simulink library "elvio"  (R2017a)
settings: Solver=VariableStepAuto  StartTime=0.0  StopTime=10.0  RelTol=1e-3
values from neighbouring files (symbols this model uses):
  Ts = 1    [dynorun.m]
  v = squeeze(v)'    [elvio_plot_scatter.m]
undefined symbols (not defined in the file or in its folder): dm, energy, F, Fmax, Fmin, Freq, m, magnitude, vcur, vref
undefined symbols (not defined in the file): containers
libraries: elvio x38, simulink x6
settings Model: Creator=elts2  LastModifiedBy=thomas

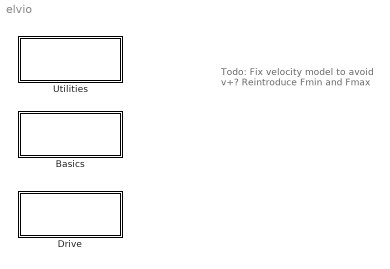
== system elvio ==
  note: Todo:
      | Fix velocity model to avoid v+?
      | Reintroduce Fmin and Fmax
  Basics : Subsystem
  Drive : Subsystem
  Utilities : Subsystem

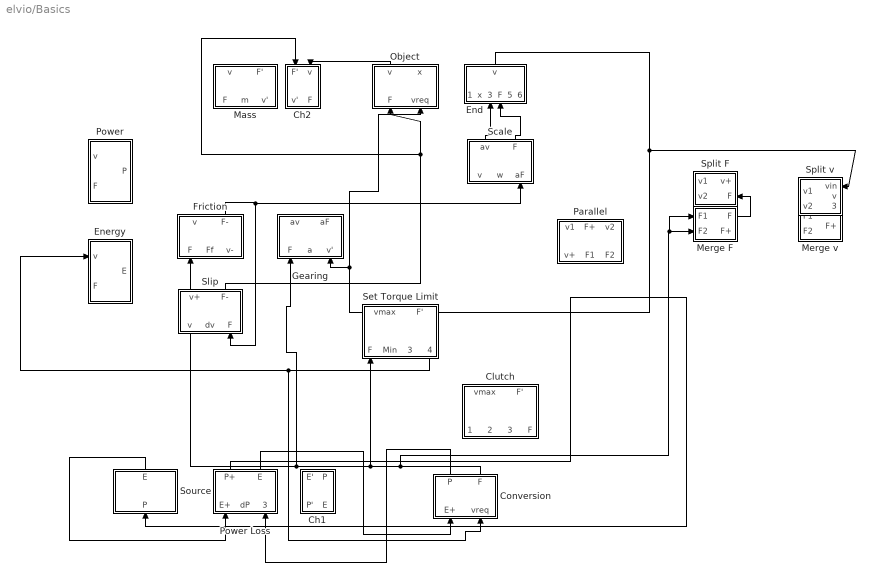
== system elvio/Basics ==
  Ch1 : Subsystem
  Ch2 : Subsystem
  Clutch : Subsystem
  Conversion : Subsystem
  End : Subsystem
  Energy : Subsystem
  Friction : Subsystem
  Gearing : Subsystem
  Mass : Subsystem
  Merge F : Subsystem
  Merge v : Subsystem
  Object : Subsystem
  Parallel : Subsystem
  Power : Subsystem
  Power Loss : Subsystem
  Scale : Subsystem
  Set Torque Limit : Subsystem
  Slip : Subsystem
  Source : Subsystem
  Split F : Subsystem
  Split v : Subsystem
  wires:
  Conversion/1(P) -> Power Loss/3(Preq)
  End/1(v) -> Split v/1(vin), Conversion/2(vreq), Energy/1(v), Object/2(vreq), Gearing/3(v')
  Power Loss/1(P+) -> Source/1(P)
  Source/1(E) -> Power Loss/1(E+)
  Conversion/2(F) -> Merge F/1(F1), Merge F/2(F2), Set Torque Limit/1(F), Gearing/1(F), Friction/1(F)
  Friction/2(F-) -> Scale/3(aF), Slip/3(F)
  Scale/1(av) -> End/3(vcur)
  Scale/2(F) -> End/4(F)
  Slip/2(F-) -> Ch2/1(F'), Object/1(F)
  Merge F/1(F) -> Split F/2(F)
  Power Loss/2(E) -> Conversion/1(E+)
  Object/1(v) -> Ch2/2(v)

== system elvio/Drive ==
  Engine : Subsystem  mask{Tmax=[40 50 60 80 100 120 150 200 300 500], Tmin=0, Tfrict=10, Ploss=1000, eff=0}
      mask prompts: Tmax "Max Torque:"; Tmin "Min Torque:"; Tfrict "Friction Torque:"; Ploss "Power Loss:"; eff "Efficiency:"
  Vehicle : Subsystem  mask{m=1200, Froll=15, Aeff=0.4, Tbrake=5000, n=[10 1]}
      mask prompts: m "Vehicle Mass:"; Froll "Tyre Friction:"; Aeff "Aero Drag:"; Tbrake "Braking Torque:"; n "Number of Simulation:"

== system elvio/Utilities ==
  Datafunction : Subsystem  mask{Cycle=NEDC, Data=[0 0 10 10 0 0]}
      mask prompts: Cycle "Driving Cycle:"; Data "Time Data:"
      mask init:
      | c=get_param(gcbh,'Cycle');
      | if c == "NEDC"
      |     set_param(gcbh,'Data','[0 0 10 10 0 0]');
      | end
      mask TypeOptions Cycle: NEDC | Artemis | FTP-75
  Display : Subsystem  StartFcn=h=add_exec_event_listener([gcb '/Display'], 'PostOutputs', @(blk,ev)set_param(gcbh,'MaskDisplay',['disp(''' num2str(blk.InputPort(1).Data) ''')']));  mask(Display the Input Value){}
      mask help: Todo: may display in the wrong blob? BUG
  Integrator : Subsystem  mask{Ts=Ts}
      mask prompts: Ts "Time Step:"
  Range : Subsystem
  Unit : Subsystem  mask(Constant value with units){Value=10, unitstr=rpm, unitmap=containers.Map({'rad/s','Hz','rpm','hrpm','krpm'},[1 2*pi 2*pi/60 2*pi/60*100 2*pi/60*1000])}
      mask prompts: Value "Simulink:blkprm_prompts:ConstConstValue"; unitmap "Unit map:"
      mask help:
      | This is a generic block for a value with units.
      |
      | The units can be configured with the field unitmap.
      mask TypeOptions Value: Constant/Value
      mask Display: disp('Value')
  Variants : Subsystem  Variant=on  VariantControl=Variant1  OverrideUsingVariant=Variant1

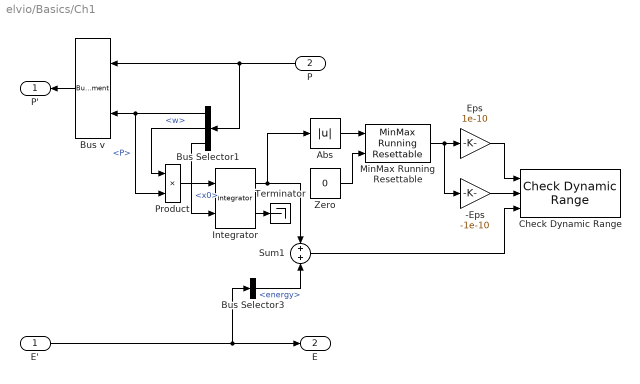
== system elvio/Basics/Ch1 ==
  E' : Inport
  P : Inport  Port=2
  -Eps : Gain  Gain=-1e-10
  Abs : Abs  ZeroCross=off
  Bus Selector1 : BusSelector  OutputSignals=P,info.w,info.x0
  Bus Selector3 : BusSelector  OutputSignals=energy
  Bus v : BusAssignment  AssignedSignals=P
  Check Dynamic Range : simulink/Model Verification/Check  Dynamic Range  Description=min < u < max  enabled=on  stopWhenAssertionFail=on  export=off  icon=graphic
      settings: SourceProductName=Simulink  SourceProductBaseCode=SL
  Eps : Gain  Gain=1e-10
  Integrator : elvio/Utilities/Integrator  Ts=Ts
  MinMax Running Resettable : simulink/Math Operations/MinMax Running Resettable  Function=max  vinit=1e-6
  Product : Product
  Sum1 : Sum
  Terminator : Terminator
  Zero : Constant  Value=0
  P' : Outport
  E : Outport  Port=2
  wires:
  Product/1 -> Integrator/1
  Bus Selector3/1 -> Sum1/2  "<energy>"
  E'/1 -> E/1, Bus Selector3/1
  Bus Selector1/3 -> Integrator/2  "<x0>"
  P/1 -> Bus Selector1/1, Bus v/1
  Bus Selector1/1 -> Bus v/2, Product/2  "<P>"
  Bus v/1 -> P'/1
  Bus Selector1/2 -> Product/1  "<w>"
  Integrator/2 -> Terminator/1
  Integrator/1 -> Abs/1, Sum1/1
  Sum1/1 -> Check Dynamic Range/3
  -Eps/1 -> Check Dynamic Range/2
  MinMax Running Resettable/1 -> -Eps/1, Eps/1
  Eps/1 -> Check Dynamic Range/1
  Zero/1 -> MinMax Running Resettable/2
  Abs/1 -> MinMax Running Resettable/1

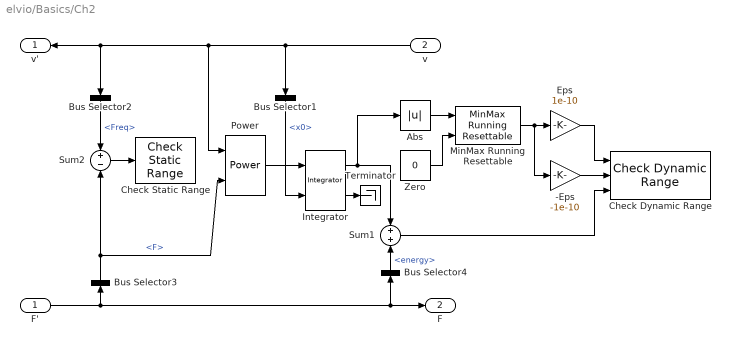
== system elvio/Basics/Ch2 ==
  F' : Inport
  v : Inport  Port=2
  -Eps : Gain  Gain=-1e-10
  Abs : Abs  ZeroCross=off
  Bus Selector1 : BusSelector  OutputSignals=info.x0
  Bus Selector2 : BusSelector  OutputSignals=Freq
  Bus Selector3 : BusSelector  OutputSignals=F
  Bus Selector4 : BusSelector  OutputSignals=energy
  Check Dynamic Range : simulink/Model Verification/Check  Dynamic Range  Description=min < u < max  enabled=on  stopWhenAssertionFail=on  export=off  icon=graphic
      settings: SourceProductName=Simulink  SourceProductBaseCode=SL
  Check Static Range : simulink/Model Verification/Check  Static Range  Description=-1e-10 <= u <= 1e-10  max=1e-10  max_included=on  min=-1e-10  min_included=on  enabled=on  stopWhenAssertionFail=on  export=off  icon=graphic
      settings: SourceProductName=Simulink  SourceProductBaseCode=SL
  Eps : Gain  Gain=1e-10
  Integrator : elvio/Utilities/Integrator  Ts=Ts
  MinMax Running Resettable : simulink/Math Operations/MinMax Running Resettable  Function=max  vinit=1e-6
  Power : elvio/Basics/Power
  Sum1 : Sum
  Sum2 : Sum  Inputs=+-
  Terminator : Terminator
  Zero : Constant  Value=0
  v' : Outport
  F : Outport  Port=2
  wires:
  Bus Selector3/1 -> Power/2, Sum2/2  "<F>"
  -Eps/1 -> Check Dynamic Range/2
  MinMax Running Resettable/1 -> -Eps/1, Eps/1
  Eps/1 -> Check Dynamic Range/1
  Abs/1 -> MinMax Running Resettable/1
  Power/1 -> Integrator/1
  Sum1/1 -> Check Dynamic Range/3
  Bus Selector4/1 -> Sum1/2  "<energy>"
  F'/1 -> F/1, Bus Selector4/1, Bus Selector3/1
  Bus Selector1/1 -> Integrator/2  "<x0>"
  v/1 -> Bus Selector1/1, Power/1, Bus Selector2/1, v'/1
  Integrator/2 -> Terminator/1
  Integrator/1 -> Sum1/1, Abs/1
  Zero/1 -> MinMax Running Resettable/2
  Bus Selector2/1 -> Sum2/1  "<Freq>"
  Sum2/1 -> Check Static Range/1

== system elvio/Basics/Clutch ==
  note: Todo
  vreq : Inport
  Fmax : Inport  Port=2
  Fmin : Inport  Port=3
  F : Inport  Port=4
  Bus Selector1 : BusSelector  OutputSignals=Freq
  Bus F : BusAssignment  AssignedSignals=Fmax,Fmin,F
  Bus v : BusAssignment  AssignedSignals=Freq
  Range : Subsystem
  vmax : Outport
  F' : Outport  Port=2
  wires:
  F/1 -> Bus F/1
  Range/1(Out) -> Bus F/4, Bus v/2  "F"
  Bus Selector1/1 -> Range/2(In)  "<Freq>"
  vreq/1 -> Bus v/1, Bus Selector1/1
  Bus v/1 -> vmax/1
  Fmin/1 -> Range/3(Min), Bus F/3  "Fmin"
  Fmax/1 -> Range/1(Max), Bus F/2
  Bus F/1 -> F'/1

== system elvio/Basics/Conversion ==
  E+ : Inport
  vreq : Inport  Port=2
  Bias1 : Bias  Bias=1e10
  Bias2 : Bias  Bias=-1e10
  Bus Creator1 : BusCreator  Inputs=8
  Bus Selector : BusSelector  OutputSignals=info.x0,Freq
  Bus Selector3 : BusSelector  OutputSignals=energy
  Constant{4..7} (4 alike) : Constant  Value=0
  Power : Subsystem
  unity : Gain
  zero : Gain  Gain=0
  P : Outport
  F : Outport  Port=2
  wires:
  Power/1(P) -> P/1
  Constant7/1 -> Bus Creator1/7  "power"
  Constant5/1 -> Bus Creator1/5  "dm"
  Bus Selector/2 -> unity/1, Power/2(F)  "<Freq>"
  Bus Creator1/1 -> F/1
  Constant6/1 -> Bus Creator1/6  "weight"
  Constant4/1 -> Bus Creator1/4  "m"
  vreq/1 -> Power/1(v), Bus Selector/1
  unity/1 -> Bus Creator1/1  "F"
  E+/1 -> Bus Selector3/1
  Bus Selector3/1 -> Bus Creator1/8  "<energy>"
  zero/1 -> Bias2/1, Bias1/1
  Bias2/1 -> Bus Creator1/3  "Fmin"
  Bus Selector/1 -> zero/1  "<x0>"
  Bias1/1 -> Bus Creator1/2  "Fmax"

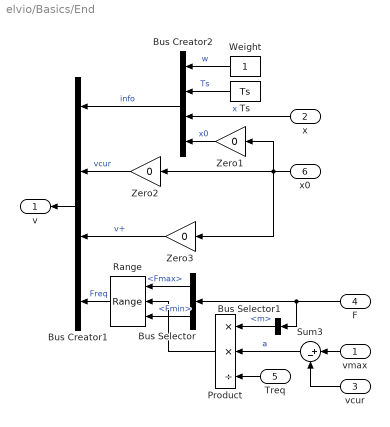
== system elvio/Basics/End ==
  vmax : Inport  Unit=m/s
  x : Inport  Port=2  Unit=m/s
  vcur : Inport  Port=3  Unit=m/s
  F : Inport  Port=4  Unit=m/s
  Treq : Inport  Port=5  Unit=m/s
  x0 : Inport  Port=6  Unit=m/s
  Bus Creator1 : BusCreator  Inputs=4
  Bus Creator2 : BusCreator  Inputs=4
  Bus Selector : BusSelector  OutputSignals=Fmax,Fmin
  Bus Selector1 : BusSelector  OutputSignals=m
  Product : Product  Inputs=**/
  Range : elvio/Utilities/Range
  Sum3 : Sum  Inputs=|+-
  Ts : Constant  Value=Ts
  Weight : Constant
  Zero1 : Gain  Gain=0
  Zero2 : Gain  Gain=0
  Zero3 : Gain  Gain=0
  v : Outport
  wires:
  x/1 -> Bus Creator2/3  "x"
  Weight/1 -> Bus Creator2/1  "w"
  Bus Creator1/1 -> v/1
  vmax/1 -> Sum3/1
  F/1 -> Bus Selector/1, Bus Selector1/1
  Bus Creator2/1 -> Bus Creator1/1  "info"
  Range/1 -> Bus Creator1/4  "Freq"
  Sum3/1 -> Product/2  "a"
  Zero2/1 -> Bus Creator1/2  "vcur"
  Zero3/1 -> Bus Creator1/3  "v+"
  vcur/1 -> Sum3/2
  Treq/1 -> Product/3
  x0/1 -> Zero2/1, Zero3/1, Zero1/1
  Zero1/1 -> Bus Creator2/4  "x0"
  Ts/1 -> Bus Creator2/2  "Ts"
  Bus Selector1/1 -> Product/1  "<m>"
  Bus Selector/1 -> Range/1  "<Fmax>"
  Bus Selector/2 -> Range/3  "<Fmin>"
  Product/1 -> Range/2

== system elvio/Basics/Energy ==
  v : Inport
  F : Inport  Port=2
  Bus Selector : BusSelector  OutputSignals=info.x0
  Integrator : elvio/Utilities/Integrator
  Power : elvio/Basics/Power
  Terminator : Terminator
  E : Outport
  wires:
  v/1 -> Bus Selector/1, Power/1
  Power/1 -> Integrator/1
  F/1 -> Power/2
  Bus Selector/1 -> Integrator/2  "<x0>"
  Integrator/2 -> Terminator/1
  Integrator/1 -> E/1

== system elvio/Basics/Friction ==
  F : Inport
  Ff : Inport  Port=2
  v- : Inport  Port=3
  Bus Selector : BusSelector  OutputSignals=F,Fmax,Fmin,energy
  Bus Selector1 : BusSelector  OutputSignals=Freq
  Bus F : BusAssignment  AssignedSignals=F,Fmax,Fmin,energy
  Bus v : BusAssignment  AssignedSignals=Freq
  Display : Display
  Energy : elvio/Basics/Energy
  Sum1 : Sum  Inputs=++|
  Sum2 : Sum  Inputs=-+|
  Sum3 : Sum  Inputs=|++
  Sum4 : Sum  Inputs=-+|
  Sum5 : Sum  Inputs=-+|
  v : Outport
  F- : Outport  Port=2
  wires:
  Energy/1 -> Display/1, Sum1/1  "E_loss_fric"
  v-/1 -> Energy/1, Bus Selector1/1, Bus v/1
  Sum3/1 -> Bus v/2  "Freq"
  Bus Selector1/1 -> Sum3/1  "<Freq>"
  Sum2/1 -> Bus F/2  "F"
  Bus F/1 -> F-/1
  Ff/1 -> Sum4/1, Sum5/1, Energy/2, Sum2/1, Sum3/2
  Bus v/1 -> v/1
  F/1 -> Bus Selector/1, Bus F/1
  Bus Selector/1 -> Sum2/2  "<F>"
  Sum1/1 -> Bus F/5
  Bus Selector/4 -> Sum1/2  "<energy>"
  Bus Selector/2 -> Sum4/2  "<Fmax>"
  Bus Selector/3 -> Sum5/2  "<Fmin>"
  Sum5/1 -> Bus F/4  "Fmin"
  Sum4/1 -> Bus F/3  "Fmax"

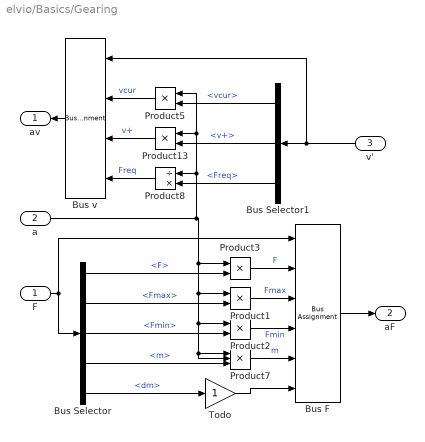
== system elvio/Basics/Gearing ==
  F : Inport
  a : Inport  Port=2
  v' : Inport  Port=3
  Bus Selector : BusSelector  OutputSignals=F,Fmax,Fmin,m,dm
  Bus Selector1 : BusSelector  OutputSignals=vcur,v+,Freq
  Bus F : BusAssignment  AssignedSignals=F,Fmax,Fmin,m,dm
  Bus v : BusAssignment  AssignedSignals=vcur,v+,Freq
  Product{1..3,5,13} (5 alike) : Product
  Product7 : Product  Inputs=***
  Product8 : Product  Inputs=/*
  Todo : Gain
  av : Outport
  aF : Outport  Port=2
  wires:
  Bus F/1 -> aF/1
  Todo/1 -> Bus F/6
  v'/1 -> Bus Selector1/1, Bus v/1
  Bus Selector1/2 -> Product13/2  "<v+>"
  Product13/1 -> Bus v/3  "v+"
  Bus Selector1/1 -> Product5/2  "<vcur>"
  F/1 -> Bus Selector/1, Bus F/1
  Product8/1 -> Bus v/4  "Freq"
  Bus v/1 -> av/1
  Bus Selector/5 -> Todo/1  "<dm>"
  Bus Selector/1 -> Product3/2  "<F>"
  Bus Selector/4 -> Product7/3  "<m>"
  a/1 -> Product8/1, Product5/1, Product13/1, Product1/1, Product2/1, Product7/2, Product7/1, Product3/1
  Product7/1 -> Bus F/5  "m"
  Product3/1 -> Bus F/2  "F"
  Bus Selector1/3 -> Product8/2  "<Freq>"
  Product5/1 -> Bus v/2  "vcur"
  Product1/1 -> Bus F/3  "Fmax"
  Bus Selector/2 -> Product1/2  "<Fmax>"
  Product2/1 -> Bus F/4  "Fmin"
  Bus Selector/3 -> Product2/2  "<Fmin>"

== system elvio/Basics/Mass ==
  F : Inport
  m : Inport  Port=2
  v' : Inport  Port=3
  Bus Assignment : BusAssignment  AssignedSignals=m
  Bus Selector : BusSelector  OutputSignals=m
  Sum : Sum  Inputs=|++
  v : Outport
  F' : Outport  Port=2
  wires:
  m/1 -> Sum/2
  Sum/1 -> Bus Assignment/2  "m"
  Bus Selector/1 -> Sum/1  "<m>"
  v'/1 -> v/1
  F/1 -> Bus Assignment/1, Bus Selector/1
  Bus Assignment/1 -> F'/1

== system elvio/Basics/Merge F ==
  F1 : Inport
  F2 : Inport  Port=2
  Bus Creator : BusCreator  Inputs=8
  Bus Selector : BusSelector  OutputSignals=F,Fmax,Fmin,m,dm,weight,power,energy
  Bus Selector2 : BusSelector  OutputSignals=F,Fmax,Fmin,m,dm,weight,power,energy
  Sum{,1..7} (8 alike) : Sum  Inputs=|++
  F : Outport
  F+ : Outport  Port=2
  wires:
  Bus Selector/6 -> Sum3/1  "<weight>"
  Bus Selector/4 -> Sum1/1  "<m>"
  Bus Selector/5 -> Sum2/1  "<dm>"
  Bus Selector/7 -> Sum4/1  "<power>"
  F1/1 -> Bus Selector/1, F/1
  Bus Selector/1 -> Sum/1  "<F>"
  F2/1 -> Bus Selector2/1
  Bus Creator/1 -> F+/1
  Sum/1 -> Bus Creator/1  "F"
  Sum2/1 -> Bus Creator/5  "dm"
  Bus Selector2/5 -> Sum2/2  "<dm>"
  Bus Selector2/1 -> Sum/2  "<F>"
  Bus Selector2/7 -> Sum4/2  "<power>"
  Sum4/1 -> Bus Creator/7  "power"
  Sum6/1 -> Bus Creator/8  "energy"
  Sum1/1 -> Bus Creator/4  "m"
  Sum3/1 -> Bus Creator/6  "weight"
  Bus Selector/8 -> Sum6/1  "<energy>"
  Bus Selector2/6 -> Sum3/2  "<weight>"
  Bus Selector2/8 -> Sum6/2  "<energy>"
  Bus Selector2/4 -> Sum1/2  "<m>"
  Bus Selector/3 -> Sum7/1  "<Fmin>"
  Sum7/1 -> Bus Creator/3  "Fmin"
  Bus Selector/2 -> Sum5/1  "<Fmax>"
  Sum5/1 -> Bus Creator/2  "Fmax"
  Bus Selector2/2 -> Sum5/2  "<Fmax>"
  Bus Selector2/3 -> Sum7/2  "<Fmin>"

== system elvio/Basics/Merge v ==
  note: Todo
  F1 : Inport
  F2 : Inport  Port=2
  Bus Creator : BusCreator  Inputs=8
  Bus Selector : BusSelector  OutputSignals=F,Fmax,Fmin,m,dm,weight,power,energy
  Bus Selector2 : BusSelector  OutputSignals=F,Fmax,Fmin,m,dm,weight,power,energy
  Highest Min : MinMax  Function=max  Inputs=2
  Lowest Max : MinMax  Inputs=2
  Sum{1..4,6} (5 alike) : Sum  Inputs=|++
  F+ : Outport
  wires:
  Bus Selector2/3 -> Highest Min/2  "<Fmin>"
  Bus Selector2/2 -> Lowest Max/2  "<Fmax>"
  Lowest Max/1 -> Bus Creator/2  "Fmax"
  Bus Selector/2 -> Lowest Max/1  "<Fmax>"
  Highest Min/1 -> Bus Creator/3  "Fmin"
  Bus Selector/3 -> Highest Min/1  "<Fmin>"
  Bus Selector2/4 -> Sum1/2  "<m>"
  Bus Selector2/8 -> Sum6/2  "<energy>"
  Bus Selector2/6 -> Sum3/2  "<weight>"
  Bus Selector/8 -> Sum6/1  "<energy>"
  Sum3/1 -> Bus Creator/6  "weight"
  Sum1/1 -> Bus Creator/4  "m"
  Sum6/1 -> Bus Creator/8  "energy"
  Sum4/1 -> Bus Creator/7  "power"
  Bus Selector2/7 -> Sum4/2  "<power>"
  Bus Selector2/5 -> Sum2/2  "<dm>"
  Sum2/1 -> Bus Creator/5  "dm"
  Bus Creator/1 -> F+/1
  F2/1 -> Bus Selector2/1
  Bus Selector/1 -> Bus Creator/1  "<F>"
  F1/1 -> Bus Selector/1
  Bus Selector/7 -> Sum4/1  "<power>"
  Bus Selector/5 -> Sum2/1  "<dm>"
  Bus Selector/4 -> Sum1/1  "<m>"
  Bus Selector/6 -> Sum3/1  "<weight>"

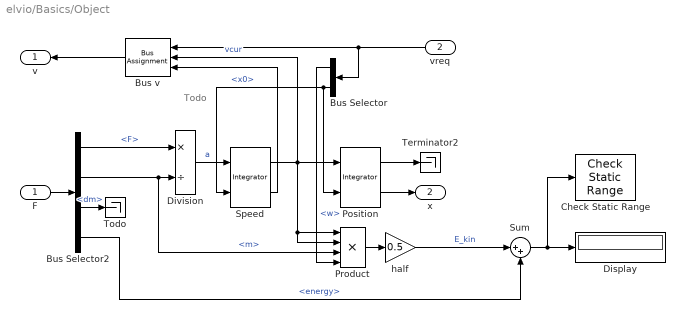
== system elvio/Basics/Object ==
  note: Todo
  F : Inport
  vreq : Inport  Port=2
  Bus Selector : BusSelector  OutputSignals=info.w,info.x0
  Bus Selector2 : BusSelector  OutputSignals=F,m,dm,energy
  Bus v : BusAssignment  AssignedSignals=vcur,v+
  Check Static Range : simulink/Model Verification/Check  Static Range  Description=-1e-3 <= u <= 1e-3  max=1e-3  max_included=on  min=-1e-3  min_included=on  enabled=on  stopWhenAssertionFail=on  export=off  icon=graphic
      settings: SourceProductName=Simulink  SourceProductBaseCode=SL
  Display : Display
  Division : Product  Inputs=*/
  Position : elvio/Utilities/Integrator  Ts=Ts
  Product : Product  Inputs=****
  Speed : elvio/Utilities/Integrator  Ts=Ts
  Sum : Sum  Inputs=|++
  Terminator2 : Terminator
  Todo : Terminator
  half : Gain  Gain=0.5
  v : Outport
  x : Outport  Port=2
  wires:
  vreq/1 -> Bus Selector/1, Bus v/1
  Bus Selector2/2 -> Product/3, Division/2  "<m>"
  Speed/1 -> Position/1, Bus v/2, Product/2, Product/1  "vcur"
  Division/1 -> Speed/1  "a"
  Product/1 -> half/1
  Bus Selector2/1 -> Division/1  "<F>"
  F/1 -> Bus Selector2/1
  half/1 -> Sum/1  "E_kin"
  Bus Selector2/3 -> Todo/1  "<dm>"
  Bus v/1 -> v/1
  Bus Selector/1 -> Product/4  "<w>"
  Position/2 -> x/1
  Position/1 -> Terminator2/1
  Speed/2 -> Bus v/3
  Bus Selector/2 -> Position/2, Speed/2  "<x0>"
  Bus Selector2/4 -> Sum/2  "<energy>"
  Sum/1 -> Check Static Range/1, Display/1

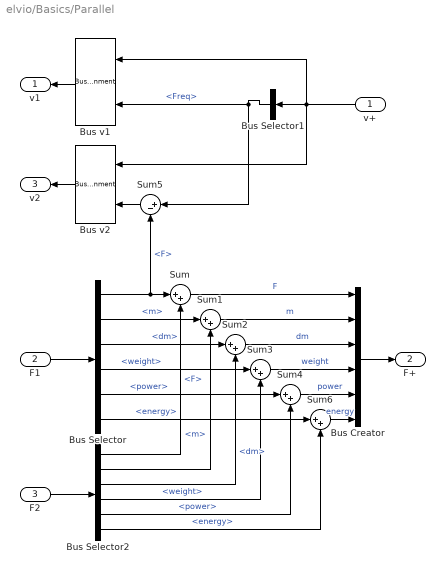
== system elvio/Basics/Parallel ==
  v+ : Inport
  F1 : Inport  Port=2
  F2 : Inport  Port=3
  Bus Creator : BusCreator  Inputs=6
  Bus Selector : BusSelector  OutputSignals=F,m,dm,weight,power,energy
  Bus Selector1 : BusSelector  OutputSignals=Freq
  Bus Selector2 : BusSelector  OutputSignals=F,m,dm,weight,power,energy
  Bus v1 : BusAssignment  AssignedSignals=Freq
  Bus v2 : BusAssignment  AssignedSignals=Freq
  Sum{,1..4,6} (6 alike) : Sum  Inputs=|++
  Sum5 : Sum  Inputs=|+-
  v1 : Outport
  F+ : Outport  Port=2
  v2 : Outport  Port=3
  wires:
  F1/1 -> Bus Selector/1
  Bus v1/1 -> v1/1
  Bus Selector1/1 -> Bus v1/2, Sum5/1  "<Freq>"
  Bus v2/1 -> v2/1
  v+/1 -> Bus v1/1, Bus v2/1, Bus Selector1/1
  Bus Selector/4 -> Sum3/1  "<weight>"
  Bus Selector/3 -> Sum2/1  "<dm>"
  Bus Selector/5 -> Sum4/1  "<power>"
  Bus Selector/2 -> Sum1/1  "<m>"
  Bus Selector/1 -> Sum5/2, Sum/1  "<F>"
  F2/1 -> Bus Selector2/1
  Bus Selector2/1 -> Sum/2  "<F>"
  Bus Selector2/2 -> Sum1/2  "<m>"
  Bus Selector2/3 -> Sum2/2  "<dm>"
  Bus Selector2/4 -> Sum3/2  "<weight>"
  Bus Selector2/5 -> Sum4/2  "<power>"
  Sum/1 -> Bus Creator/1  "F"
  Sum1/1 -> Bus Creator/2  "m"
  Sum2/1 -> Bus Creator/3  "dm"
  Sum3/1 -> Bus Creator/4  "weight"
  Sum4/1 -> Bus Creator/5  "power"
  Bus Creator/1 -> F+/1
  Sum5/1 -> Bus v2/2
  Sum6/1 -> Bus Creator/6  "energy"
  Bus Selector2/6 -> Sum6/2  "<energy>"
  Bus Selector/6 -> Sum6/1  "<energy>"

== system elvio/Basics/Power ==
  v : Inport
  F : Inport  Port=2
  Bus Selector2 : BusSelector  OutputSignals=vcur,v+,info.w
  Product : Product  Inputs=***
  Sum4 : Sum  Inputs=++|
  half : Gain  Gain=0.5
  P : Outport
  wires:
  half/1 -> P/1
  Bus Selector2/3 -> Product/2  "<w>"
  Bus Selector2/2 -> Sum4/2  "<v+>"
  Bus Selector2/1 -> Sum4/1  "<vcur>"
  F/1 -> Product/3
  v/1 -> Bus Selector2/1
  Sum4/1 -> Product/1
  Product/1 -> half/1

== system elvio/Basics/Power Loss ==
  E+ : Inport
  dP : Inport  Port=2
  Preq : Inport  Port=3
  Bus Selector1 : BusSelector  OutputSignals=P,info.w,info.x0
  Bus Selector3 : BusSelector  OutputSignals=energy
  Bus E : BusAssignment  AssignedSignals=energy
  Bus v : BusAssignment  AssignedSignals=P
  Display : Display
  Integrator : elvio/Utilities/Integrator  Ts=Ts
  Product : Product
  Sum1 : Sum  Inputs=++|
  Sum3 : Sum  Inputs=|++
  Terminator : Terminator
  P+ : Outport
  E : Outport  Port=2
  wires:
  Integrator/1 -> Sum1/1, Display/1  "E_power_loss"
  Integrator/2 -> Terminator/1
  Product/1 -> Integrator/1
  Bus Selector1/2 -> Product/1  "<w>"
  Bus v/1 -> P+/1
  Bus Selector1/1 -> Sum3/1  "<P>"
  Sum3/1 -> Bus v/2  "Freq"
  dP/1 -> Sum3/2, Product/2
  Preq/1 -> Bus v/1, Bus Selector1/1
  Bus Selector1/3 -> Integrator/2  "<x0>"
  E+/1 -> Bus Selector3/1, Bus E/1
  Sum1/1 -> Bus E/2
  Bus E/1 -> E/1
  Bus Selector3/1 -> Sum1/2  "<energy>"

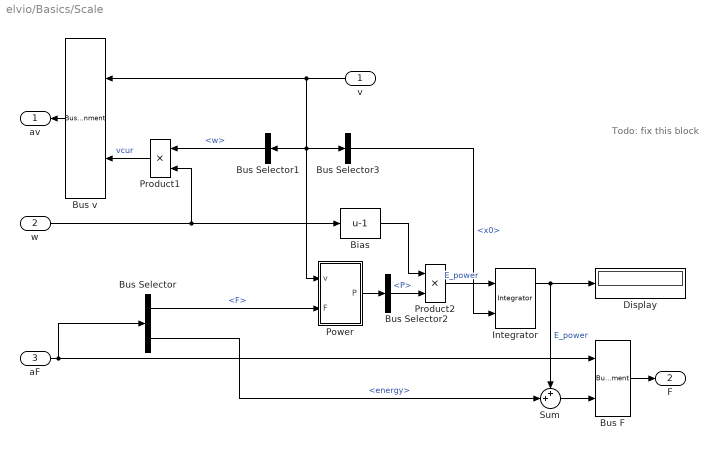
== system elvio/Basics/Scale ==
  note: Todo: fix this block
  v : Inport
  w : Inport  Port=2
  aF : Inport  Port=3
  Bias : Bias  Bias=-1
  Bus Selector : BusSelector  OutputSignals=F,energy
  Bus Selector1 : BusSelector  OutputSignals=info.w
  Bus Selector2 : BusSelector  OutputSignals=P
  Bus Selector3 : BusSelector  OutputSignals=info.x0
  Bus F : BusAssignment  AssignedSignals=energy
  Bus v : BusAssignment  AssignedSignals=info.w
  Display : Display
  Integrator : elvio/Utilities/Integrator  Ts=Ts
  Power : Subsystem
  Product1 : Product
  Product2 : Product
  Sum : Sum  Inputs=++|
  av : Outport
  F : Outport  Port=2
  wires:
  Integrator/1 -> Sum/1, Display/1  "E_power"
  Bus Selector3/1 -> Integrator/2  "<x0>"
  Product2/1 -> Integrator/1  "E_power"
  Bias/1 -> Product2/1
  w/1 -> Product1/2, Bias/1
  Bus Selector2/1 -> Product2/2  "<P>"
  Bus Selector/1 -> Power/2(F)  "<F>"
  v/1 -> Bus v/1, Bus Selector1/1, Power/1(v), Bus Selector3/1
  Power/1(P) -> Bus Selector2/1
  Product1/1 -> Bus v/2  "vcur"
  Bus v/1 -> av/1
  Bus Selector1/1 -> Product1/1  "<w>"
  aF/1 -> Bus Selector/1, Bus F/1
  Bus F/1 -> F/1
  Sum/1 -> Bus F/2
  Bus Selector/2 -> Sum/2  "<energy>"

== system elvio/Basics/Set Torque Limit ==
  F : Inport
  Min : Inport  Port=2
  Max : Inport  Port=3
  vreq : Inport  Port=4
  Bus Selector : BusSelector  OutputSignals=Freq
  Bus Selector1 : BusSelector  OutputSignals=Fmax,Fmin
  Bus F : BusAssignment  AssignedSignals=Fmax,Fmin
  Bus v : BusAssignment  AssignedSignals=Freq
  Highest Min : MinMax  Function=max  Inputs=2
  Lowest Max : MinMax  Inputs=2
  Range : elvio/Utilities/Range
  vmax : Outport
  F' : Outport  Port=2
  wires:
  F/1 -> Bus Selector1/1, Bus F/1
  Bus v/1 -> vmax/1
  vreq/1 -> Bus Selector/1, Bus v/1
  Range/1 -> Bus v/2
  Bus Selector/1 -> Range/2  "<Freq>"
  Bus F/1 -> F'/1
  Lowest Max/1 -> Range/1, Bus F/2
  Highest Min/1 -> Range/3, Bus F/3
  Bus Selector1/1 -> Lowest Max/2  "<Fmax>"
  Bus Selector1/2 -> Highest Min/2  "<Fmin>"
  Max/1 -> Lowest Max/1
  Min/1 -> Highest Min/1

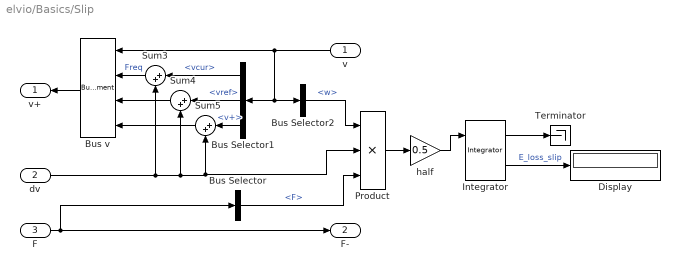
== system elvio/Basics/Slip ==
  v : Inport
  dv : Inport  Port=2
  F : Inport  Port=3
  Bus Selector : BusSelector  OutputSignals=F
  Bus Selector1 : BusSelector  OutputSignals=vcur,vref,v+
  Bus Selector2 : BusSelector  OutputSignals=info.w
  Bus v : BusAssignment  AssignedSignals=vcur,vref,v+
  Display : Display
  Integrator : elvio/Utilities/Integrator  Ts=Ts
  Product : Product  Inputs=***
  Sum3 : Sum  Inputs=|++
  Sum4 : Sum  Inputs=|++
  Sum5 : Sum  Inputs=|++
  Terminator : Terminator
  half : Gain  Gain=0.5
  v+ : Outport
  F- : Outport  Port=2
  wires:
  Bus Selector2/1 -> Product/1  "<w>"
  v/1 -> Bus v/1, Bus Selector1/1, Bus Selector2/1
  half/1 -> Integrator/1
  Bus Selector/1 -> Product/3  "<F>"
  Integrator/2 -> Display/1  "E_loss_slip"
  Product/1 -> half/1
  dv/1 -> Sum3/2, Sum5/2, Product/2, Sum4/2
  Integrator/1 -> Terminator/1
  Sum5/1 -> Bus v/4
  Bus Selector1/2 -> Sum4/1  "<vref>"
  Bus Selector1/3 -> Sum5/1  "<v+>"
  Sum4/1 -> Bus v/3
  Sum3/1 -> Bus v/2  "Freq"
  Bus Selector1/1 -> Sum3/1  "<vcur>"
  F/1 -> Bus Selector/1, F-/1
  Bus v/1 -> v+/1

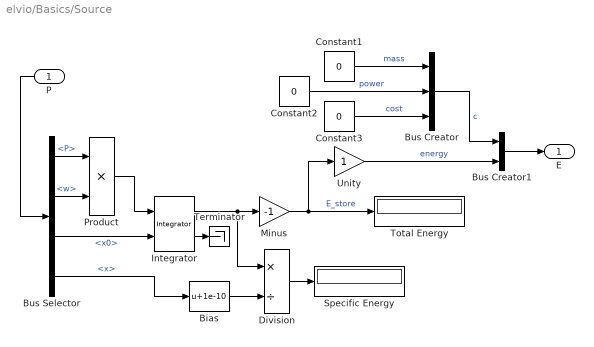
== system elvio/Basics/Source ==
  P : Inport
  Bias : Bias  Bias=1e-10
  Bus Creator : BusCreator  Inputs=3
  Bus Creator1 : BusCreator  Inputs=2
  Bus Selector : BusSelector  OutputSignals=P,info.w,info.x0,info.x
  Constant1 : Constant  Value=0
  Constant2 : Constant  Value=0
  Constant3 : Constant  Value=0
  Division : Product  Inputs=*/
  Integrator : elvio/Utilities/Integrator  Ts=Ts
  Minus : Gain  Gain=-1
  Product : Product  Inputs=**
  Specific Energy : Display
  Terminator : Terminator
  Total Energy : Display
  Unity : Gain
  E : Outport
  wires:
  Integrator/2 -> Terminator/1
  Minus/1 -> Unity/1, Total Energy/1  "E_store"
  Product/1 -> Integrator/1
  P/1 -> Bus Selector/1
  Bus Selector/1 -> Product/1  "<P>"
  Bus Selector/2 -> Product/2  "<w>"
  Bus Selector/4 -> Bias/1  "<x>"
  Division/1 -> Specific Energy/1
  Bus Selector/3 -> Integrator/2  "<x0>"
  Integrator/1 -> Minus/1, Division/1
  Unity/1 -> Bus Creator1/2  "energy"
  Bus Creator/1 -> Bus Creator1/1  "c"
  Bus Creator1/1 -> E/1
  Constant1/1 -> Bus Creator/1  "mass"
  Constant3/1 -> Bus Creator/3  "cost"
  Constant2/1 -> Bus Creator/2  "power"
  Bias/1 -> Division/2

== system elvio/Basics/Split F ==
  v+ : Inport
  F : Inport  Port=2
  Bus Selector : BusSelector  OutputSignals=F,Fmax,Fmin
  Bus Selector1 : BusSelector  OutputSignals=Freq
  Bus v1 : BusAssignment  AssignedSignals=Freq
  Bus v2 : BusAssignment  AssignedSignals=Freq
  Range : elvio/Utilities/Range
  Sum5 : Sum  Inputs=|+-
  v1 : Outport
  v2 : Outport  Port=2
  wires:
  Bus v2/1 -> v2/1
  Bus v1/1 -> v1/1
  Bus Selector1/1 -> Range/2, Sum5/1  "<Freq>"
  v+/1 -> Bus v2/1, Bus v1/1, Bus Selector1/1
  Sum5/1 -> Bus v2/2
  F/1 -> Bus Selector/1
  Bus Selector/1 -> Sum5/2  "<F>"
  Range/1 -> Bus v1/2
  Bus Selector/2 -> Range/1  "<Fmax>"
  Bus Selector/3 -> Range/3  "<Fmin>"

== system elvio/Basics/Split v ==
  vin : Inport
  v : Inport  Port=2
  v+1 : Inport  Port=3
  Bus Selector1 : BusSelector  OutputSignals=vcur,v+
  Bus v1 : BusAssignment  AssignedSignals=vcur,v+
  Bus v2 : BusAssignment  AssignedSignals=vcur,v+
  Sum1 : Sum  Inputs=-+|
  Sum5 : Sum  Inputs=-+|
  v1 : Outport
  v2 : Outport  Port=2
  wires:
  v/1 -> Bus v1/2, Sum5/1
  Sum5/1 -> Bus v2/2
  vin/1 -> Bus v2/1, Bus Selector1/1, Bus v1/1
  Bus Selector1/1 -> Sum5/2  "<vcur>"
  Bus v1/1 -> v1/1
  Bus v2/1 -> v2/1
  Sum1/1 -> Bus v2/3
  v+1/1 -> Sum1/1, Bus v1/3
  Bus Selector1/2 -> Sum1/2  "<v+>"

== system elvio/Drive/Engine ==
  E : Inport
  vreq : Inport  Port=2
  Aux Loss : Constant  Value=Ploss
  Ch1 : elvio/Basics/Ch2
  Ch2 : elvio/Basics/Ch2
  Ch3 : elvio/Basics/Ch1
  Conv : elvio/Basics/Conversion
  Force Limit : elvio/Basics/Set Torque Limit
  Friction : elvio/Basics/Friction
  Friction Torque : Constant  Value=Tfrict
  Max Tqrue : Constant  Value=Tmax
  Min Torque : Constant  Value=Tmin
  Power Loss : elvio/Basics/Power Loss
  Sum : Sum  Inputs=|-+
  P : Outport
  F : Outport  Port=2
  wires:
  Min Torque/1 -> Sum/2
  Friction Torque/1 -> Sum/1, Friction/2
  Force Limit/2 -> F/1
  vreq/1 -> Force Limit/4
  Friction/2 -> Ch2/1
  Sum/1 -> Force Limit/2
  Aux Loss/1 -> Power Loss/2
  Max Tqrue/1 -> Force Limit/3
  Ch3/2 -> Conv/1
  Conv/1 -> Ch3/2
  Force Limit/1 -> Ch2/2
  Ch2/1 -> Friction/3
  Ch2/2 -> Force Limit/1
  Power Loss/1 -> P/1
  Power Loss/2 -> Ch3/1
  Ch3/1 -> Power Loss/3
  Conv/2 -> Ch1/1
  Friction/1 -> Ch1/2
  Ch1/2 -> Friction/1
  Ch1/1 -> Conv/2
  E/1 -> Power Loss/1

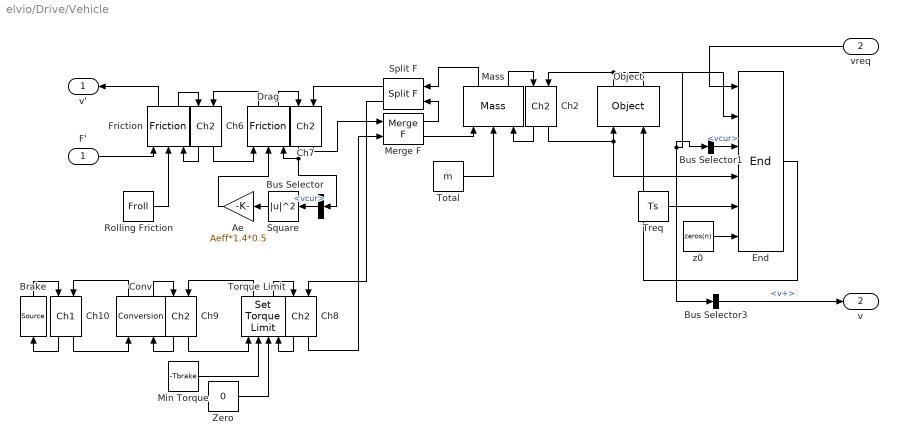
== system elvio/Drive/Vehicle ==
  F' : Inport
  vreq : Inport  Port=2
  Ae : Gain  Gain=Aeff*1.4*0.5
  Brake : elvio/Basics/Source
  Bus Selector : BusSelector  OutputSignals=vcur
  Bus Selector1 : BusSelector  OutputSignals=vcur
  Bus Selector3 : BusSelector  OutputSignals=v+
  Ch10 : elvio/Basics/Ch1
  Ch{2,6..9} (5 alike) : elvio/Basics/Ch2
  Conv : elvio/Basics/Conversion
  Drag : elvio/Basics/Friction
  End : elvio/Basics/End
  Friction : elvio/Basics/Friction
  Mass : elvio/Basics/Mass
  Merge F : elvio/Basics/Merge F
  Min Torque : Constant  Value=-Tbrake
  Object : elvio/Basics/Object
  Rolling Friction : Constant  Value=Froll
  Split F : elvio/Basics/Split F
  Square : Math  Operator=magnitude^2  SaturateOnIntegerOverflow=on
  Torque Limit : elvio/Basics/Set Torque Limit
  Total : Constant  Value=m
  Treq : Constant  Value=Ts
  Zero : Constant  Value=0
  z0 : Constant  Value=zeros(n)
  v' : Outport
  v : Outport  Port=2
  wires:
  Torque Limit/1 -> Ch9/2
  Square/1 -> Ae/1
  Ae/1 -> Drag/2
  Total/1 -> Mass/2
  Bus Selector/1 -> Square/1  "<vcur>"
  Mass/1 -> Split F/1
  Split F/2 -> Ch8/2
  Min Torque/1 -> Torque Limit/2
  Merge F/2 -> Mass/1
  Ch8/2 -> Merge F/2
  Zero/1 -> Torque Limit/3
  Ch9/2 -> Torque Limit/1
  Ch7/1 -> Drag/3, Bus Selector/1
  Split F/1 -> Ch7/2
  Ch9/1 -> Conv/2
  Ch7/2 -> Merge F/1
  Torque Limit/2 -> Ch8/1
  Ch6/2 -> Drag/1
  Friction/1 -> v'/1
  Ch10/2 -> Conv/1
  Conv/2 -> Ch9/1
  Merge F/1 -> Split F/2
  Drag/2 -> Ch7/1
  Ch8/1 -> Torque Limit/4
  Brake/1 -> Ch10/1
  Ch10/1 -> Brake/1
  Conv/1 -> Ch10/2
  Ch6/1 -> Friction/3
  F'/1 -> Friction/1
  Friction/2 -> Ch6/1
  Rolling Friction/1 -> Friction/2
  Drag/1 -> Ch6/2
  Object/2 -> End/2
  End/1 -> Object/2
  Treq/1 -> End/5
  Bus Selector3/1 -> v/1  "<v+>"
  z0/1 -> End/6
  Bus Selector1/1 -> End/3  "<vcur>"
  vreq/1 -> End/1
  Ch2/2 -> End/4, Object/1
  Object/1 -> Ch2/2, Bus Selector1/1, Bus Selector3/1
  Mass/2 -> Ch2/1
  Ch2/1 -> Mass/3

== system elvio/Utilities/Datafunction ==
  In1 : Inport
  1-D Lookup Table : Lookup_n-D  NumberOfTableDimensions=1  BreakpointsForDimension1=[0:2:10]  Table=Data  InternalRulePriority=Speed  RndMeth=Simplest  InputSameDT=on
  Out1 : Outport
  wires:
  1-D Lookup Table/1 -> Out1/1
  In1/1 -> 1-D Lookup Table/1

== system elvio/Utilities/Display ==
  In1 : Inport
  Display : Display
  wires:
  In1/1 -> Display/1

== system elvio/Utilities/Integrator ==
  dx : Inport
  x0 : Inport  Port=2
  Delay : Delay  DelayLength=1  InitialConditionSource=Input port  SampleTime=abs(Ts)
      settings: InputPortMap=u0,p4
  Product : Product
  Sum5 : Sum  Inputs=|++
  Ts : Constant  Value=Ts
  x : Outport
  x+ : Outport  Port=2
  wires:
  Sum5/1 -> Delay/1, x+/1
  Delay/1 -> Sum5/2, x/1
  Product/1 -> Sum5/1
  dx/1 -> Product/1
  Ts/1 -> Product/2
  x0/1 -> Delay/2

== system elvio/Utilities/Range ==
  Max : Inport
  In : Inport  Port=2
  Min : Inport  Port=3
  MinMax1 : MinMax  Inputs=2
  MinMax2 : MinMax  Function=max  Inputs=2
  Out : Outport
  wires:
  MinMax1/1 -> MinMax2/1  "F"
  In/1 -> MinMax1/1
  MinMax2/1 -> Out/1  "F"
  Min/1 -> MinMax2/2
  Max/1 -> MinMax1/2

== system elvio/Utilities/Unit ==
  Constant : Constant  Value=Value
  Unit : Gain  Gain=unitmap(unitstr)
  Out : Outport
  wires:
  Constant/1 -> Unit/1
  Unit/1 -> Out/1

== system elvio/Utilities/Variants ==
  "In1 " : Inport
  Double : Subsystem  VariantControl=Variant
  Subsystem : Subsystem  VariantControl=Variant1
  " Out1" : Outport

== system elvio/Basics/Clutch/Range ==
  Max : Inport
  In : Inport  Port=2
  Min : Inport  Port=3
  MinMax1 : MinMax  Inputs=2
  MinMax2 : MinMax  Function=max  Inputs=2
  Out : Outport
  wires:
  MinMax1/1 -> MinMax2/1  "F"
  In/1 -> MinMax1/1
  MinMax2/1 -> Out/1  "F"
  Min/1 -> MinMax2/2
  Max/1 -> MinMax1/2

== system elvio/Basics/Conversion/Power ==
  v : Inport
  F : Inport  Port=2
  Bus Creator : BusCreator  Inputs=2
  Bus Selector1 : BusSelector  OutputSignals=info
  Bus Selector2 : BusSelector  OutputSignals=vcur,v+
  Product : Product  Inputs=**
  Sum4 : Sum
  half : Gain  Gain=0.5
  P : Outport
  wires:
  Product/1 -> half/1
  Sum4/1 -> Product/1
  v/1 -> Bus Selector1/1, Bus Selector2/1
  F/1 -> Product/2
  Bus Selector2/1 -> Sum4/1  "<vcur>"
  Bus Selector2/2 -> Sum4/2  "<v+>"
  Bus Selector1/1 -> Bus Creator/2  "<info>"
  Bus Creator/1 -> P/1
  half/1 -> Bus Creator/1  "P"

== system elvio/Basics/Scale/Power ==
  v : Inport
  F : Inport  Port=2
  Bus Creator : BusCreator  Inputs=2
  Bus Selector1 : BusSelector  OutputSignals=info
  Bus Selector2 : BusSelector  OutputSignals=vcur,v+
  Product : Product  Inputs=**
  Sum4 : Sum
  half : Gain  Gain=0.5
  P : Outport
  wires:
  half/1 -> Bus Creator/1  "P"
  Bus Creator/1 -> P/1
  Bus Selector1/1 -> Bus Creator/2  "<info>"
  Bus Selector2/2 -> Sum4/2  "<v+>"
  Bus Selector2/1 -> Sum4/1  "<vcur>"
  F/1 -> Product/2
  v/1 -> Bus Selector2/1, Bus Selector1/1
  Sum4/1 -> Product/1
  Product/1 -> half/1

== system elvio/Utilities/Variants/Double ==
  "In1 " : Inport
  Gain : Gain
  " Out1" : Outport
  wires:
  "In1 "/1 -> Gain/1
  Gain/1 -> " Out1"/1

== system elvio/Utilities/Variants/Subsystem ==
  In1 : Inport
  Gain : Gain
  Out1 : Outport
  wires:
  In1/1 -> Gain/1
  Gain/1 -> Out1/1
